simulink model "SBW_SystemModel"  (R2019b)
settings: Solver=ode1  StartTime=0.0  StopTime=3  FixedStep=0.001  RelTol=1e-3  EnableMultiTasking=on
PostLoadFcn:
  | , if any(exist('dsrtsu_mdlpostloadfcn', 'file') == [2, 3, 6]), try dsrtsu_mdlpostloadfcn('Execute', bdroot); catch fprintf('Error in PostLoadFcn (dsrtsu_mdlpostloadfcn) for model "%s":\n %s\n', bdroot, lasterr); end, end,
values from neighbouring files (symbols this model uses):
  B = 0.51    [SBW_main.m]    (also in Single_Obj_pso.m; multi_obj_fminimax.m; multi_obj_mopso.m; singleObjFunc.m)
  J = 0.1475    [SBW_main.m]    (also in Single_Obj_pso.m; multi_obj_fminimax.m; multi_obj_mopso.m; singleObjFunc.m)
  Tf = 2.2613    [SBW_main.m]    (also in Single_Obj_pso.m; multi_obj_fminimax.m; multi_obj_mopso.m; singleObjFunc.m)
  x = [200,1,20,0,0]    [SBW_main.m]    (also in Single_Obj_pso.m = abs(x) .*[1000, 10, 100,1,1]; multi_obj_mopso.m = abs(x) .*[1000, 10, 100,1,1]; single_obj_fminsearch.m = OrderedList(); single_obj_nelder_and_mead.m = zeros(nrParam,nrParam+1))
undefined symbols (not defined in the file or in its folder): magnitude
libraries: powerlib_meascontrol x2, simulink x1
settings Model: DSRTSU_INTERNAL_RTI_VER=460  DSRTSU_INTERNAL_RTI_TYPE=rti1401  RTICANMMDATA=struct('GeneralSetupData',struct('modelroot',['C:\Users\ECLab\Desktop\Simulation 358'],'generalsettings',struct('filesettings',struct('destfolder',struct('Name','RTICANMM_FILES','Check',1),'buildfolder',struct('Name','.','Check',1),'AbsDestfolder',struct('Name',['C:\Users\ECLab\Desktop\Simulation 358\RTICANMM_FILES']),'AbsBuildfolder',struct('Name',['C:\Users\ECLab\Desktop\Simulation 358']))),'options',struct('addpaths',1,'rmpaths',1,'addtrcexclusion',logical(1),'cannavigator',struct('checkmonitoring',0),'show_usrtrc',0,'use_usrtrc',0),'advanced',struct('options',[1 1 1 1 1 1 1 1 1 1 1 1 1 1 1 1 1 1 1 1 1 1 1 1 1 1 1 1 1 1 1 1 1 1 1 1 1 1 1 1 1 1 1 1 1 1 1 1 1 1 1 1 1 1 1 1 1 1 1 1 1 1 1 1 1 1 1 1 1 1 1 1 1 1 1 1 1 1 1 1 1 1 1 1 1 1 1 1 1 1 1 1 1 1 1 1 1 1 1 1]),'MPSetup',{{}},'modelname','SBW','block','SBW'))  DSRTSU_INTERNAL_RTIFLEXRAYCONFIG=80  DSRTSU_INTERNAL_RTIFPGA=50  Creator=ECLab  LastModifiedBy=wouter
settings DataIOCC: LimitDataPoints=on  SaveFormat=Array  ReturnWorkspaceOutputs=off
settings OptimizationCC: BlockReduction=off  OptimizeBlockIOStorage=off  BufferReuse=off  GlobalBufferReuse=off  ExpressionFolding=off  LocalBlockOutputs=off  LifeSpan=inf  OptimizeDataStoreBuffers=off  BusAssignmentInplaceUpdate=off
settings DebuggingCC: UnderspecifiedInitializationDetection=Classic  MergeDetectMultiDrivingBlocksExec=none  MaxConsecutiveZCsMsg=none  SolverPrmCheckMsg=warning  SFUnexpectedBacktrackingDiag=warning  SFNoUnconditionalDefaultTransitionDiag=warning  SFExecutionAtInitializationDiag=none  ArithmeticOperatorsInVariantConditions=warning
settings HardwareCC: ProdBitPerPointer=32  ProdBitPerSizeT=32  ProdBitPerPtrDiffT=32  ProdLargestAtomicFloat=None  ProdEndianess=BigEndian  ProdWordSize=32  ProdHWDeviceType=Generic->Custom  TargetIntDivRoundTo=Zero  TargetEndianess=BigEndian  TargetHWDeviceType=Generic->Custom
settings ModelReferenceCC: PropagateSignalLabelsOutOfModel=off
settings SFSimCC: SimUseLocalCustomCode=off  CustomCodeUndefinedFunction=UseInterfaceOnly
settings RTWCC: Description=dSPACE DS1401 Hardware Platform  SystemTargetFile=rti1401.tlc  MakeCommand=make_rti  TemplateMakefile=rti1401.tmf  RTWUseLocalCustomCode=off
settings CodeAppCC: StateflowObjectComments=on
settings STFCustomTargetCC: ParMdlRefBuildCompliant=on  GeneratePreprocessorConditionals=Disable all  MatFileLogging=on  CPPClassGenCompliant=on  GRTInterface=on  SystemTargetFile=rti1401.tlc
settings GRTTargetCC: TargetLangStandard=C89/C90 (ANSI)  CompOptLevelCompliant=off  ConcurrentExecutionCompliant=off  GeneratePreprocessorConditionals=Disable all  CombineOutputUpdateFcns=off  GRTInterface=on  UseToolchainInfoCompliant=off  ExtModeMexFile=noextcomm
settings ConfigComp: CovMetricSettings=dw  CovHtmlReporting=on  CovSaveCumulativeToWorkspaceVar=on  CovSaveSingleToWorkspaceVar=on  CovExternalEMLEnable=off

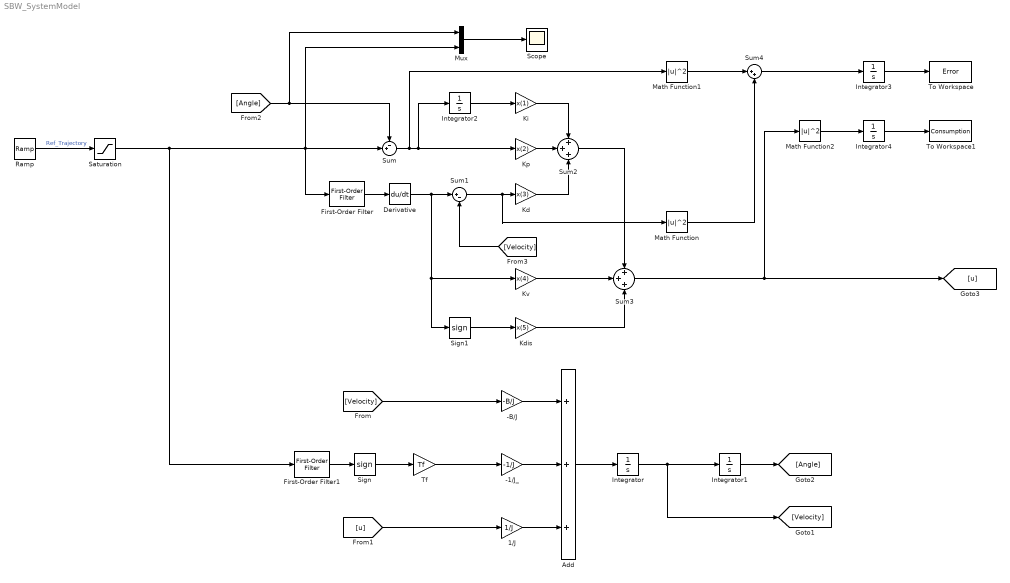
== system SBW_SystemModel ==
  -1/J_ : Gain  Gain=-1/J
  -B/J : Gain  Gain=-B/J
  1/J : Gain  Gain=1/J
  Add : Sum  Inputs=+++
  Derivative : Derivative
  First-Order Filter : powerlib_meascontrol/Filters/First-Order Filter  FilterType=Lowpass  Tc=10e-3  Ts=0  Initialize=on  Vac_Init=[0, 0, 60]  Vdc_Init=0  PlotResponse=off  FreqRange="[0,  200,  1]"
      settings: SourceProductName=Simscape Electrical
  First-Order Filter1 : powerlib_meascontrol/Filters/First-Order Filter  FilterType=Lowpass  Tc=10e-3  Ts=0  Initialize=on  Vac_Init=[0, 0, 60]  Vdc_Init=0  PlotResponse=off  FreqRange="[0,  200,  1]"
      settings: SourceProductName=Simscape Electrical
  Integrator{,1..4} (5 alike) : Integrator
  Kd : Gain  Gain=x(3)
  Kdis : Gain  Gain=x(5)
  Ki : Gain  Gain=x(1)
  Kp : Gain  Gain=x(2)
  Kv : Gain  Gain=x(4)
  Math Function : Math  Operator=magnitude^2  SaturateOnIntegerOverflow=on
  Math Function1 : Math  Operator=magnitude^2  SaturateOnIntegerOverflow=on
  Math Function2 : Math  Operator=magnitude^2  SaturateOnIntegerOverflow=on
  Mux : Mux  Inputs=2
  Ramp : simulink/Sources/Ramp  slope=pi/2  start=0  InitialOutput=0
  Saturation : Saturate  UpperLimit=pi/2  LowerLimit=0
  Scope : Scope
  Sign : Signum
  Sign1 : Signum
  Sum : Sum  Inputs=-+|
  Sum1 : Sum  Inputs=|+-
  Sum2 : Sum  Inputs=+++
  Sum3 : Sum  Inputs=+++
  Sum4 : Sum  Inputs=|++
  Tf : Gain  Gain=Tf
  To Workspace : ToWorkspace  VariableName=Error  SampleTime=-1
  To Workspace1 : ToWorkspace  VariableName=Consumption  SampleTime=-1
  wires:
  Kd/1 -> Sum2/3
  Integrator2/1 -> Ki/1
  First-Order Filter/1 -> Derivative/1
  Saturation/1 -> First-Order Filter1/1, Mux/2, First-Order Filter/1, Sum/2
  [u] -> 1/J/1
  [Angle] -> Mux/1, Sum/1
  Ramp/1 -> Saturation/1  "Ref_Trajectory"
  Sum1/1 -> Math Function/1, Kd/1
  Tf/1 -> -1/J_/1
  [Velocity] -> -B/J/1
  [Velocity] -> Sum1/2
  Sum/1 -> Math Function1/1, Integrator2/1, Kp/1
  Ki/1 -> Sum2/1
  Add/1 -> Integrator/1
  Derivative/1 -> Sign1/1, Kv/1, Sum1/1
  Integrator/1 -> [Velocity], Integrator1/1
  1/J/1 -> Add/3
  -B/J/1 -> Add/1
  Integrator1/1 -> [Angle]
  Sum3/1 -> [u], Math Function2/1
  Kdis/1 -> Sum3/3
  Kv/1 -> Sum3/2
  Kp/1 -> Sum2/2
  Sign1/1 -> Kdis/1
  First-Order Filter1/1 -> Sign/1
  -1/J_/1 -> Add/2
  Sum2/1 -> Sum3/1
  Mux/1 -> Scope/1
  Sign/1 -> Tf/1
  Math Function/1 -> Sum4/2
  Math Function1/1 -> Sum4/1
  Sum4/1 -> Integrator3/1
  Integrator3/1 -> To Workspace/1
  Integrator4/1 -> To Workspace1/1
  Math Function2/1 -> Integrator4/1
